simulink model "Lab2"  (R2023b)
settings: Solver=VariableStepAuto  StartTime=0.0  StopTime=0.02  RelTol=1e-3
libraries: spsVoltageMeasurementLib x4, spsACVoltageSourceLib x3, spsRMSLib x3, spsSeriesRLCBranchLib x3, spsGroundLib x2, eePowerMeasurement x2, spsCurrentMeasurementLib x1, spsThreePhaseVIMeasurementLib x1, sps_lib x1
settings Model: Creator=Shreetej  LastModifiedBy=Shreetej

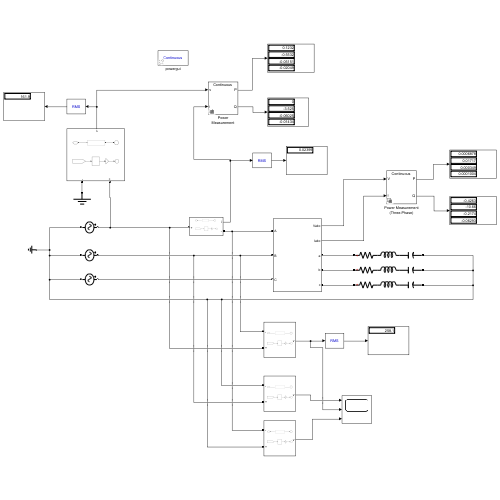
[thumbnail: Simulink's stored preview of the top-level diagram]
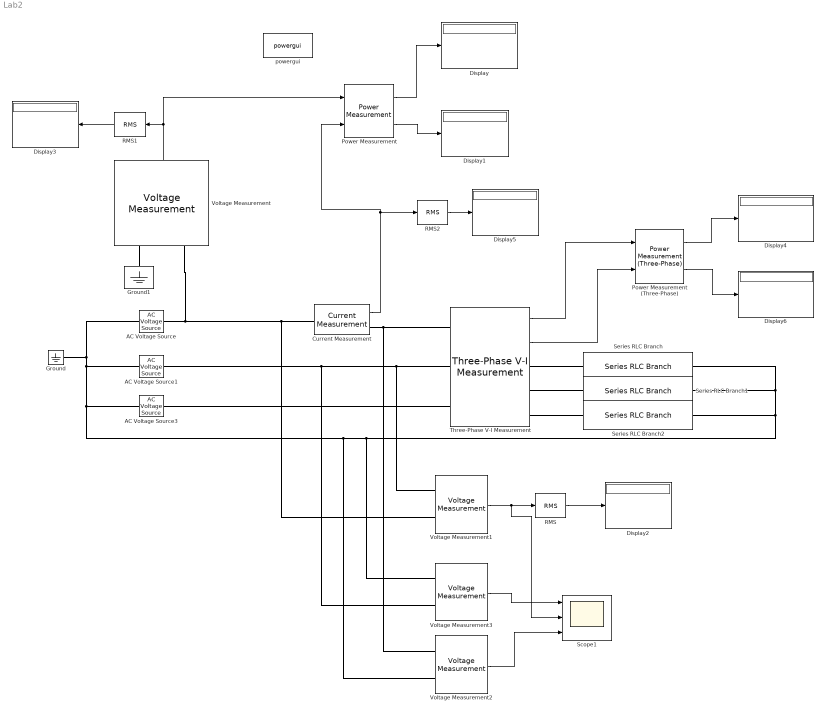
== system Lab2 ==
  AC Voltage Source : spsACVoltageSourceLib/AC Voltage Source  Amplitude=220  Phase=0  Frequency=50  SampleTime=0  Measurements=None  BusType=swing  Pref=10e3  Qref=0  Qmin=-inf  Qmax=+inf
  AC Voltage Source1 : spsACVoltageSourceLib/AC Voltage Source  Amplitude=220  Phase=-120  Frequency=50  SampleTime=0  Measurements=None  BusType=swing  Pref=10e3  Qref=0  Qmin=-inf  Qmax=+inf
  AC Voltage Source3 : spsACVoltageSourceLib/AC Voltage Source  Amplitude=220  Phase=-240  Frequency=50  SampleTime=0  Measurements=None  BusType=swing  Pref=10e3  Qref=0  Qmin=-inf  Qmax=+inf
  Current Measurement : spsCurrentMeasurementLib/Current Measurement  PhasorSimulation=off  OutputType=Complex  PSBequivalent=0
  Display{,1..6} (7 alike) : Display
      Display settings: Decimation=2
      Display4 settings: Decimation=2
      Display6 settings: Decimation=2
  Ground : spsGroundLib/Ground  LConnTagsString=a
  Ground1 : spsGroundLib/Ground  LConnTagsString=a
  Power Measurement : eePowerMeasurement/Power Measurement  LabelModeActiveChoice=Continuous  F=60  K=[0 1 2 3]  Ts=0
  Power Measurement (Three-Phase) : eePowerMeasurement/Power Measurement (Three-Phase)  LabelModeActiveChoice=Continuous  F=60  K=[0 1 2 3]  Seq=Positive  Ts=0
  RMS : spsRMSLib/RMS  TrueRMS=on  Freq=60  RMSInit=120  Ts=0
  RMS1 : spsRMSLib/RMS  TrueRMS=on  Freq=60  RMSInit=120  Ts=0
  RMS2 : spsRMSLib/RMS  TrueRMS=on  Freq=60  RMSInit=120  Ts=0
  Scope1 : Scope  NumInputPorts=3
  Series RLC Branch : spsSeriesRLCBranchLib/Series RLC Branch  LConnTagsString=__new0  RConnTagsString=__new0  BranchType=RLC  Resistance=10  Inductance=0.5  SetiL0=off  InitialCurrent=0  Capacitance=0.5e-6  Setx0=off  InitialVoltage=0  Measurements=None
  Series RLC Branch1 : spsSeriesRLCBranchLib/Series RLC Branch  LConnTagsString=__new0  RConnTagsString=__new0  BranchType=RLC  Resistance=10  Inductance=0.5  SetiL0=off  InitialCurrent=0  Capacitance=0.5e-6  Setx0=off  InitialVoltage=0  Measurements=None
  Series RLC Branch2 : spsSeriesRLCBranchLib/Series RLC Branch  LConnTagsString=__new0  RConnTagsString=__new0  BranchType=RLC  Resistance=10  Inductance=0.5  SetiL0=off  InitialCurrent=0  Capacitance=0.5e-6  Setx0=off  InitialVoltage=0  Measurements=None
  Three-Phase V-I Measurement : spsThreePhaseVIMeasurementLib/Three-Phase V-I Measurement  VoltageMeasurement=phase-to-ground  SetLabelV=off  LabelV=Vabc  Vpu=off  VpuLL=off  CurrentMeasurement=yes  SetLabelI=off  LabelI=Iabc  Ipu=off  Pbase=100e6  Vbase=500e3  OutputType=Complex  PhasorSimulation=off  PSBequivalent=0
  Voltage Measurement{,1..3} (4 alike) : spsVoltageMeasurementLib/Voltage Measurement  PhasorSimulation=off  OutputType=Complex  PSBequivalent=0
  powergui : sps_lib/powergui  Priority=1  SimulationMode=Continuous  SampleTime=50e-6  frequency=60  Iterations=50  frequencyindice=50  Pbase=100e6  ErrMax=1e-4  UnitsV=kV  UnitsW=MW  buscounter=0  FunctionMessages=off  echomessages=off  EnableUseOfTLC=off  CurrentSourceSwitches=off  DisableSnubberDevices=off  DisableRonSwitches=off  DisableVfSwitches=off  DisplayEquations=off  AutomaticDiscreteSolvers=off  SolverType=Tustin/Backward Euler (TBE)  Interpol=off  ExternalGateDelay=off  methode=off  Ts=100  x0status=blocks  SPID=on  SwTol=0  HookPort=off  NonlinearTolerance=1e-4  nMaxIteration=100  ContinueOnMaxIteration=off  RestoreLinks=warning  ResistiveCurrentMeasurement=off  Frange=[0:2:500]  Ylog=off  Xlog=on  ShowGrid=off  save=off  variable=ZData  structure=0  ZoomFFT=off  StartTime=0.0  cycles=1  DisplayStyle=1  fundamental=60  FreqAxis=off  MaxFrequency=1000  frequencyindicesteady=1  RmsSteady=1  display=off
  wires:
  Power Measurement/1 -> Display/1
  Voltage Measurement/1 -> RMS1/1, Power Measurement/1
  Current Measurement/1 -> Power Measurement/2, RMS2/1
  Power Measurement/2 -> Display1/1
  Three-Phase V-I Measurement/1 -> Power Measurement (Three-Phase)/1
  Three-Phase V-I Measurement/2 -> Power Measurement (Three-Phase)/2
  Power Measurement (Three-Phase)/1 -> Display4/1
  Power Measurement (Three-Phase)/2 -> Display6/1
  RMS1/1 -> Display3/1
  RMS2/1 -> Display5/1
  Voltage Measurement3/1 -> Scope1/1
  Voltage Measurement2/1 -> Scope1/3
  RMS/1 -> Display2/1
  Voltage Measurement1/1 -> RMS/1, Scope1/2
  connections:
  AC Voltage Source1/LConn1 -- AC Voltage Source/LConn1 -- Ground/LConn1 -- AC Voltage Source3/LConn1 -- Voltage Measurement2/LConn1 -- Voltage Measurement3/LConn2 -- Series RLC Branch/RConn1 -- Series RLC Branch1/RConn1 -- Series RLC Branch2/RConn1
  Voltage Measurement/LConn1 -- Voltage Measurement1/LConn1 -- Current Measurement/LConn1 -- AC Voltage Source/RConn1
  AC Voltage Source1/RConn1 -- Voltage Measurement3/LConn1 -- Three-Phase V-I Measurement/LConn2 -- Voltage Measurement1/LConn2
  Current Measurement/RConn1 -- Three-Phase V-I Measurement/LConn1 -- Voltage Measurement2/LConn2
  AC Voltage Source3/RConn1 -- Three-Phase V-I Measurement/LConn3
  Three-Phase V-I Measurement/RConn1 -- Series RLC Branch/LConn1
  Three-Phase V-I Measurement/RConn2 -- Series RLC Branch1/LConn1
  Three-Phase V-I Measurement/RConn3 -- Series RLC Branch2/LConn1
  Ground1/LConn1 -- Voltage Measurement/LConn2
